simulink model "gm_gmStateSpaceHDL_uz_JL_invModel_ideal"  (R2025a)
settings: Solver=FixedStepDiscrete  StartTime=0.0  StopTime=0.1  RelTol=1e-3
InitFcn:
  | load('C:\Users\jonat\Nextcloud\Ohm\ELSYS\MA_Jonathan_Link\Simulink\sschdl\uz_JL_invModel_ideal\stateSpaceParameters.mat');
undefined symbols (not defined in the file or in its folder): stateSpaceParameters_1
libraries: hdlmdlgenlib x7, hdlssclib x2
settings Model: Creator=jonat  LastModifiedBy=jonat
settings SolverCC: AlgebraicLoopSolver=TrustRegion
settings DataIOCC: LimitDataPoints=on  SaveOutput=off  SaveTime=off
settings OptimizationCC: BlockReduction=off  ConditionallyExecuteInputs=off  DefaultParameterBehavior=Inlined  InheritOutputTypeSmallerThanSingle=on  LifeSpan=inf
settings DebuggingCC: AlgebraicLoopMsg=error  InheritedTsInSrcMsg=none  SingleTaskRateTransMsg=error  UnconnectedInputMsg=warning  UnconnectedOutputMsg=warning  UnconnectedLineMsg=warning  AllowSymbolicDim=off  StrictBusMsg=ErrorOnBusTreatedAsVector  SFUnexpectedBacktrackingDiag=warning  SFNoUnconditionalDefaultTransitionDiag=warning  SFExecutionAtInitializationDiag=none  ArithmeticOperatorsInVariantConditions=warning
settings HardwareCC: ProdBitPerPointer=32.0  ProdBitPerSizeT=32.0  ProdBitPerPtrDiffT=32.0  ProdLargestAtomicFloat=None  ProdIntDivRoundTo=Undefined  ProdEndianess=Unspecified  ProdWordSize=32.0  ProdHWDeviceType=ASIC/FPGA->ASIC/FPGA  ProdEqTarget=off
settings ModelReferenceCC: EnableRefExpFcnMdlSchedulingChecks=on
settings SFSimCC: SimUseLocalCustomCode=off  CustomCodeUndefinedFunction=UseInterfaceOnly
settings RTWCC: RTWUseLocalCustomCode=off  GPUComputeCapability=3.5
settings CodeAppCC: StateflowObjectComments=on
settings GRTTargetCC: TargetLangStandard=C89/C90 (ANSI)
settings ConfigComp: CovScope=ReferencedModels  CovMetricSettings=dw  CovSaveCumulativeToWorkspaceVar=on  CovSaveSingleToWorkspaceVar=on  CovExternalEMLEnable=off  CovSFcnEnable=off

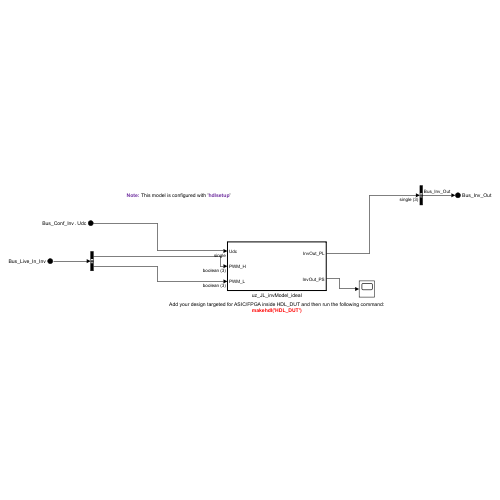
[thumbnail: Simulink's stored preview of the top-level diagram]
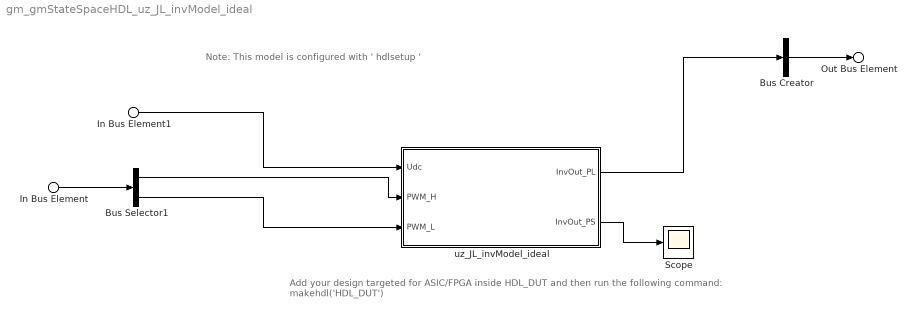
== system gm_gmStateSpaceHDL_uz_JL_invModel_ideal ==
  note: Add your design targeted for ASIC/FPGA inside HDL_DUT and then run the following command:
      | makehdl('HDL_DUT')
  note: Note: This model is configured with ' hdlsetup '
  In Bus Element : Inport  PortName=Bus_Live_In_Inv
  In Bus Element1 : Inport  Port=2  PortName=Bus_Conf_Inv  Element=Udc
  Bus Creator : BusCreator  Inputs=1  OutDataTypeStr=Bus: Bus_Inv_Out  NonVirtualBus=on
      settings: InheritFromInputs=off
  Bus Selector1 : BusSelector  OutputSignals=PWM_H,PWM_L
  Scope : Scope
      settings: ActiveDisplayYMinimum=-497.00837732959218  ActiveDisplayYMaximum=484.07881017040796
  uz_JL_invModel_ideal : Subsystem  TreatAsAtomicUnit=on
  Out Bus Element : Outport  PortName=Bus_Inv_Out
  wires:
  uz_JL_invModel_ideal/1(InvOut_PL) -> Bus Creator/1
  Bus Selector1/2 -> uz_JL_invModel_ideal/3(PWM_L)
  Bus Selector1/1 -> uz_JL_invModel_ideal/2(PWM_H)
  In Bus Element1/1 -> uz_JL_invModel_ideal/1(Udc)
  uz_JL_invModel_ideal/2(InvOut_PS) -> Scope/1
  Bus Creator/1 -> Out Bus Element/1
  In Bus Element/1 -> Bus Selector1/1

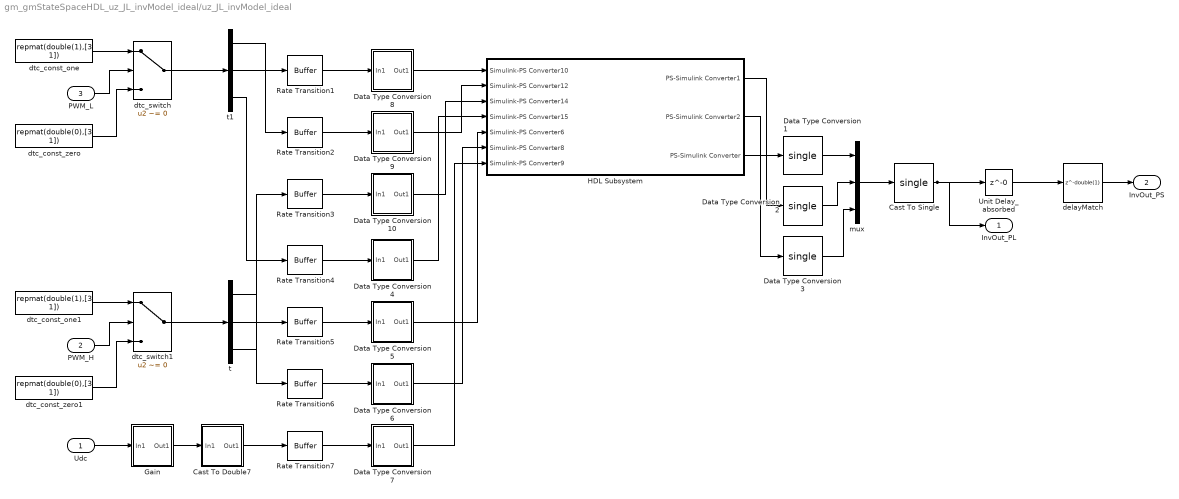
== system gm_gmStateSpaceHDL_uz_JL_invModel_ideal/uz_JL_invModel_ideal ==
  Udc : Inport  OutDataTypeStr=single  PortDimensions=1  SampleTime=1e-08
  PWM_H : Inport  Port=2  OutDataTypeStr=boolean  PortDimensions=[3]  SampleTime=1e-08
  PWM_L : Inport  Port=3  OutDataTypeStr=boolean  PortDimensions=[3]  SampleTime=1e-08
  Cast To Double7 : Subsystem
      mask Display: disp('NFP\nconv');
  Cast To Single : DataTypeConversion  OutDataTypeStr=single
  Data Type Conversion1 : DataTypeConversion  OutDataTypeStr=single
  Data Type Conversion10 : Subsystem
      mask Display: disp('NFP\nconv');
  Data Type Conversion2 : DataTypeConversion  OutDataTypeStr=single
  Data Type Conversion3 : DataTypeConversion  OutDataTypeStr=single
  Data Type Conversion4 : Subsystem
      mask Display: disp('NFP\nconv');
  Data Type Conversion5 : Subsystem
      mask Display: disp('NFP\nconv');
  Data Type Conversion6 : Subsystem
      mask Display: disp('NFP\nconv');
  Data Type Conversion7 : Subsystem
      mask Display: disp('NFP\nconv');
  Data Type Conversion8 : Subsystem
      mask Display: disp('NFP\nconv');
  Data Type Conversion9 : Subsystem
      mask Display: disp('NFP\nconv');
  Gain : Subsystem
      mask Display: disp('NFP\ngain_pow2');
  HDL Subsystem : Subsystem
  Rate Transition{1..7} (7 alike) : hdlmdlgenlib/Buffer
  Unit Delay_absorbed : Delay  DelayLength=0
  delayMatch : Delay  DelayLength=double(1)  InitialCondition=0  SampleTime=1e-08
  dtc_const_one : Constant  Value="repmat(double(1),[3  1])"  OutDataTypeStr=double  SampleTime=1e-08
  dtc_const_one1 : Constant  Value="repmat(double(1),[3  1])"  OutDataTypeStr=double  SampleTime=1e-08
  dtc_const_zero : Constant  Value="repmat(double(0),[3  1])"  OutDataTypeStr=double  SampleTime=1e-08
  dtc_const_zero1 : Constant  Value="repmat(double(0),[3  1])"  OutDataTypeStr=double  SampleTime=1e-08
  dtc_switch : Switch  Criteria=u2 ~= 0  Threshold=double(0)  OutDataTypeStr=double  SampleTime=1e-08  SaturateOnIntegerOverflow=off  InputSameDT=off
  dtc_switch1 : Switch  Criteria=u2 ~= 0  Threshold=double(0)  OutDataTypeStr=double  SampleTime=1e-08  SaturateOnIntegerOverflow=off  InputSameDT=off
  mux : Mux  Inputs=3
  t : Demux  Outputs=3
  t1 : Demux  Outputs=3
  InvOut_PL : Outport  SampleTime=1e-08
  InvOut_PS : Outport  Port=2  SampleTime=1e-08
  wires:
  dtc_const_one/1 -> dtc_switch/1
  dtc_const_one1/1 -> dtc_switch1/1
  delayMatch/1 -> InvOut_PS/1
  PWM_L/1 -> dtc_switch/2
  dtc_const_zero/1 -> dtc_switch/3
  dtc_const_zero1/1 -> dtc_switch1/3
  PWM_H/1 -> dtc_switch1/2
  Data Type Conversion4/1(Out1) -> HDL Subsystem/4(Simulink-PS Converter15)
  Data Type Conversion8/1(Out1) -> HDL Subsystem/1(Simulink-PS Converter10)
  dtc_switch/1 -> t1/1
  Udc/1 -> Gain/1(In1)
  dtc_switch1/1 -> t/1
  Data Type Conversion5/1(Out1) -> HDL Subsystem/5(Simulink-PS Converter6)
  Data Type Conversion9/1(Out1) -> HDL Subsystem/2(Simulink-PS Converter12)
  Gain/1(Out1) -> Cast To Double7/1(In1)
  Data Type Conversion7/1(Out1) -> HDL Subsystem/7(Simulink-PS Converter9)
  Data Type Conversion10/1(Out1) -> HDL Subsystem/3(Simulink-PS Converter14)
  t1/1 -> Rate Transition2/1
  HDL Subsystem/1(PS-Simulink Converter1) -> Data Type Conversion2/1
  t1/2 -> Rate Transition1/1
  t1/3 -> Rate Transition4/1
  t/1 -> Rate Transition6/1
  t/2 -> Rate Transition5/1
  t/3 -> Rate Transition3/1
  Data Type Conversion6/1(Out1) -> HDL Subsystem/6(Simulink-PS Converter8)
  Cast To Double7/1(Out1) -> Rate Transition7/1
  Rate Transition1/1 -> Data Type Conversion8/1(In1)
  Rate Transition2/1 -> Data Type Conversion9/1(In1)
  Rate Transition3/1 -> Data Type Conversion10/1(In1)
  Rate Transition4/1 -> Data Type Conversion4/1(In1)
  Rate Transition5/1 -> Data Type Conversion5/1(In1)
  Rate Transition6/1 -> Data Type Conversion6/1(In1)
  HDL Subsystem/2(PS-Simulink Converter2) -> Data Type Conversion3/1
  Rate Transition7/1 -> Data Type Conversion7/1(In1)
  HDL Subsystem/3(PS-Simulink Converter) -> Data Type Conversion1/1
  Data Type Conversion1/1 -> mux/1
  Data Type Conversion2/1 -> mux/2
  Data Type Conversion3/1 -> mux/3
  mux/1 -> Cast To Single/1
  Unit Delay_absorbed/1 -> delayMatch/1
  Cast To Single/1 -> InvOut_PL/1, Unit Delay_absorbed/1

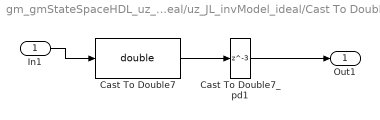
== system gm_gmStateSpaceHDL_uz_JL_invModel_ideal/uz_JL_invModel_ideal/Cast To Double7 ==
  In1 : Inport
  Cast To Double7 : DataTypeConversion  OutDataTypeStr=double  SampleTime=1e-08  SaturateOnIntegerOverflow=off  RndMeth=Floor
  Cast To Double7_pd1 : Delay  DelayLength=3
  Out1 : Outport
  wires:
  In1/1 -> Cast To Double7/1
  Cast To Double7/1 -> Cast To Double7_pd1/1
  Cast To Double7_pd1/1 -> Out1/1

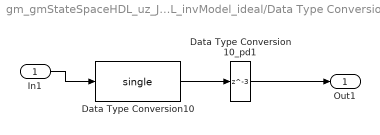
== system gm_gmStateSpaceHDL_uz_JL_invModel_ideal/uz_JL_invModel_ideal/Data Type Conversion10 ==
  In1 : Inport
  Data Type Conversion10 : DataTypeConversion  OutDataTypeStr=single  RndMeth=Nearest  SampleTime=1e-08  SaturateOnIntegerOverflow=off
  Data Type Conversion10_pd1 : Delay  DelayLength=3
  Out1 : Outport
  wires:
  In1/1 -> Data Type Conversion10/1
  Data Type Conversion10/1 -> Data Type Conversion10_pd1/1
  Data Type Conversion10_pd1/1 -> Out1/1

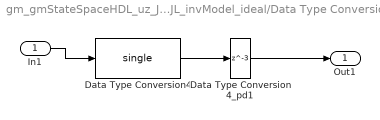
== system gm_gmStateSpaceHDL_uz_JL_invModel_ideal/uz_JL_invModel_ideal/Data Type Conversion4 ==
  In1 : Inport
  Data Type Conversion4 : DataTypeConversion  OutDataTypeStr=single  RndMeth=Nearest  SampleTime=1e-08  SaturateOnIntegerOverflow=off
  Data Type Conversion4_pd1 : Delay  DelayLength=3
  Out1 : Outport
  wires:
  In1/1 -> Data Type Conversion4/1
  Data Type Conversion4/1 -> Data Type Conversion4_pd1/1
  Data Type Conversion4_pd1/1 -> Out1/1

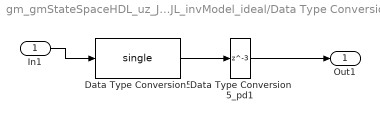
== system gm_gmStateSpaceHDL_uz_JL_invModel_ideal/uz_JL_invModel_ideal/Data Type Conversion5 ==
  In1 : Inport
  Data Type Conversion5 : DataTypeConversion  OutDataTypeStr=single  RndMeth=Nearest  SampleTime=1e-08  SaturateOnIntegerOverflow=off
  Data Type Conversion5_pd1 : Delay  DelayLength=3
  Out1 : Outport
  wires:
  In1/1 -> Data Type Conversion5/1
  Data Type Conversion5/1 -> Data Type Conversion5_pd1/1
  Data Type Conversion5_pd1/1 -> Out1/1

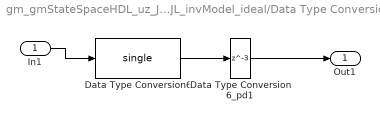
== system gm_gmStateSpaceHDL_uz_JL_invModel_ideal/uz_JL_invModel_ideal/Data Type Conversion6 ==
  In1 : Inport
  Data Type Conversion6 : DataTypeConversion  OutDataTypeStr=single  RndMeth=Nearest  SampleTime=1e-08  SaturateOnIntegerOverflow=off
  Data Type Conversion6_pd1 : Delay  DelayLength=3
  Out1 : Outport
  wires:
  In1/1 -> Data Type Conversion6/1
  Data Type Conversion6/1 -> Data Type Conversion6_pd1/1
  Data Type Conversion6_pd1/1 -> Out1/1

== system gm_gmStateSpaceHDL_uz_JL_invModel_ideal/uz_JL_invModel_ideal/Data Type Conversion7 ==
  In1 : Inport
  Data Type Conversion7 : DataTypeConversion  OutDataTypeStr=single  RndMeth=Nearest  SampleTime=1e-08  SaturateOnIntegerOverflow=off
  Data Type Conversion7_pd1 : Delay  DelayLength=3
  Out1 : Outport
  wires:
  In1/1 -> Data Type Conversion7/1
  Data Type Conversion7/1 -> Data Type Conversion7_pd1/1
  Data Type Conversion7_pd1/1 -> Out1/1

== system gm_gmStateSpaceHDL_uz_JL_invModel_ideal/uz_JL_invModel_ideal/Data Type Conversion8 ==
  In1 : Inport
  Data Type Conversion8 : DataTypeConversion  OutDataTypeStr=single  RndMeth=Nearest  SampleTime=1e-08  SaturateOnIntegerOverflow=off
  Data Type Conversion8_pd1 : Delay  DelayLength=3
  Out1 : Outport
  wires:
  In1/1 -> Data Type Conversion8/1
  Data Type Conversion8/1 -> Data Type Conversion8_pd1/1
  Data Type Conversion8_pd1/1 -> Out1/1

== system gm_gmStateSpaceHDL_uz_JL_invModel_ideal/uz_JL_invModel_ideal/Data Type Conversion9 ==
  In1 : Inport
  Data Type Conversion9 : DataTypeConversion  OutDataTypeStr=single  RndMeth=Nearest  SampleTime=1e-08  SaturateOnIntegerOverflow=off
  Data Type Conversion9_pd1 : Delay  DelayLength=3
  Out1 : Outport
  wires:
  In1/1 -> Data Type Conversion9/1
  Data Type Conversion9/1 -> Data Type Conversion9_pd1/1
  Data Type Conversion9_pd1/1 -> Out1/1

== system gm_gmStateSpaceHDL_uz_JL_invModel_ideal/uz_JL_invModel_ideal/Gain ==
  In1 : Inport
  Gain : Gain  Gain=single(0.5)
  Gain_pd1 : Delay  DelayLength=1
  Out1 : Outport
  wires:
  In1/1 -> Gain/1
  Gain/1 -> Gain_pd1/1
  Gain_pd1/1 -> Out1/1

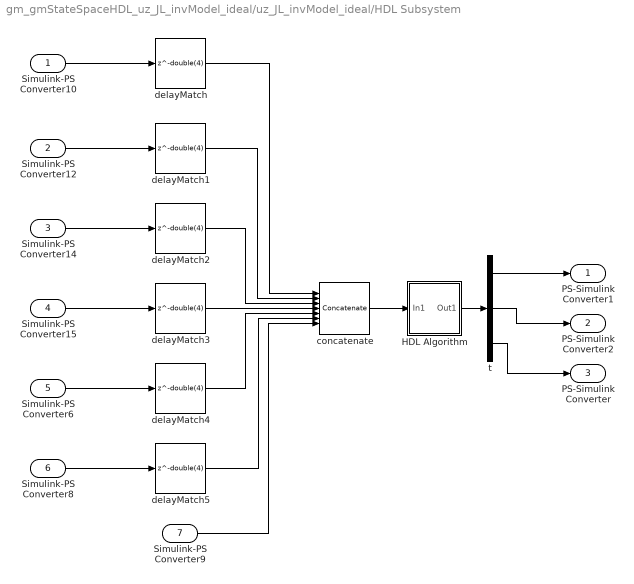
== system gm_gmStateSpaceHDL_uz_JL_invModel_ideal/uz_JL_invModel_ideal/HDL Subsystem ==
  Simulink-PS Converter10 : Inport  OutDataTypeStr=single  PortDimensions=1  SampleTime=1e-08
  Simulink-PS Converter12 : Inport  Port=2  OutDataTypeStr=single  PortDimensions=1  SampleTime=1e-08
  Simulink-PS Converter14 : Inport  Port=3  OutDataTypeStr=single  PortDimensions=1  SampleTime=1e-08
  Simulink-PS Converter15 : Inport  Port=4  OutDataTypeStr=single  PortDimensions=1  SampleTime=1e-08
  Simulink-PS Converter6 : Inport  Port=5  OutDataTypeStr=single  PortDimensions=1  SampleTime=1e-08
  Simulink-PS Converter8 : Inport  Port=6  OutDataTypeStr=single  PortDimensions=1  SampleTime=1e-08
  Simulink-PS Converter9 : Inport  Port=7  OutDataTypeStr=single  PortDimensions=1  SampleTime=1e-08
  HDL Algorithm : Subsystem
  concatenate : Concatenate  NumInputs=7
  delayMatch{,1..5} (6 alike) : Delay  DelayLength=double(4)  InitialCondition=0  SampleTime=1e-08
  t : Demux  Outputs=3
  PS-Simulink Converter1 : Outport  SampleTime=1e-08
  PS-Simulink Converter2 : Outport  Port=2  SampleTime=1e-08
  PS-Simulink Converter : Outport  Port=3  SampleTime=1e-08
  wires:
  Simulink-PS Converter6/1 -> delayMatch4/1
  Simulink-PS Converter10/1 -> delayMatch/1
  Simulink-PS Converter8/1 -> delayMatch5/1
  Simulink-PS Converter12/1 -> delayMatch1/1
  Simulink-PS Converter14/1 -> delayMatch2/1
  t/3 -> PS-Simulink Converter/1
  Simulink-PS Converter15/1 -> delayMatch3/1
  delayMatch/1 -> concatenate/1
  delayMatch1/1 -> concatenate/2
  delayMatch2/1 -> concatenate/3
  delayMatch3/1 -> concatenate/4
  delayMatch4/1 -> concatenate/5
  delayMatch5/1 -> concatenate/6
  Simulink-PS Converter9/1 -> concatenate/7
  t/1 -> PS-Simulink Converter1/1
  concatenate/1 -> HDL Algorithm/1(In1)
  HDL Algorithm/1(Out1) -> t/1
  t/2 -> PS-Simulink Converter2/1

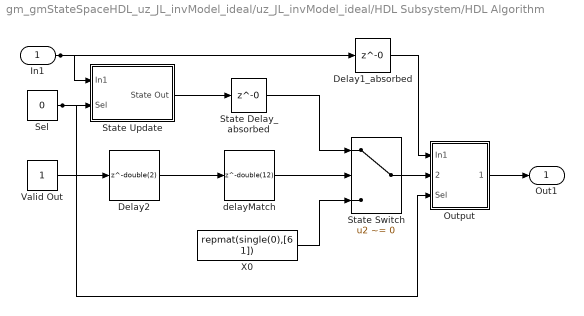
== system gm_gmStateSpaceHDL_uz_JL_invModel_ideal/uz_JL_invModel_ideal/HDL Subsystem/HDL Algorithm ==
  In1 : Inport  OutDataTypeStr=single  PortDimensions=[7]  SampleTime=1e-08
  Delay1_absorbed : Delay  DelayLength=0
  Delay2 : Delay  DelayLength=double(2)  InitialCondition=0  SampleTime=1e-08
  Output : Subsystem
  Sel : Constant  Value=0  OutDataTypeStr=uint32  SampleTime=1e-08
  State Delay_absorbed : Delay  DelayLength=0
  State Switch : Switch  Criteria=u2 ~= 0  Threshold="fi(0,0,1,0,\"hex\",\"0\")"  OutDataTypeStr=single  SampleTime=1e-08  SaturateOnIntegerOverflow=off  InputSameDT=off
  State Update : Subsystem
  Valid Out : Constant  OutDataTypeStr=boolean  SampleTime=1e-08
  X0 : Constant  Value="repmat(single(0),[6  1])"  OutDataTypeStr=single  SampleTime=1e-08
  delayMatch : Delay  DelayLength=double(12)  InitialCondition=0  SampleTime=1e-08
  Out1 : Outport  SampleTime=1e-08  VectorParamsAs1DForOutWhenUnconnected=off
  wires:
  In1/1 -> Delay1_absorbed/1, State Update/1(In1)
  X0/1 -> State Switch/3
  delayMatch/1 -> State Switch/2
  Sel/1 -> Output/3(Sel), State Update/2(Sel)
  State Delay_absorbed/1 -> State Switch/1
  Valid Out/1 -> Delay2/1
  State Update/1(State Out) -> State Delay_absorbed/1
  Delay2/1 -> delayMatch/1
  Delay1_absorbed/1 -> Output/1(In1)
  State Switch/1 -> Output/2(State)
  Output/1(Out1) -> Out1/1

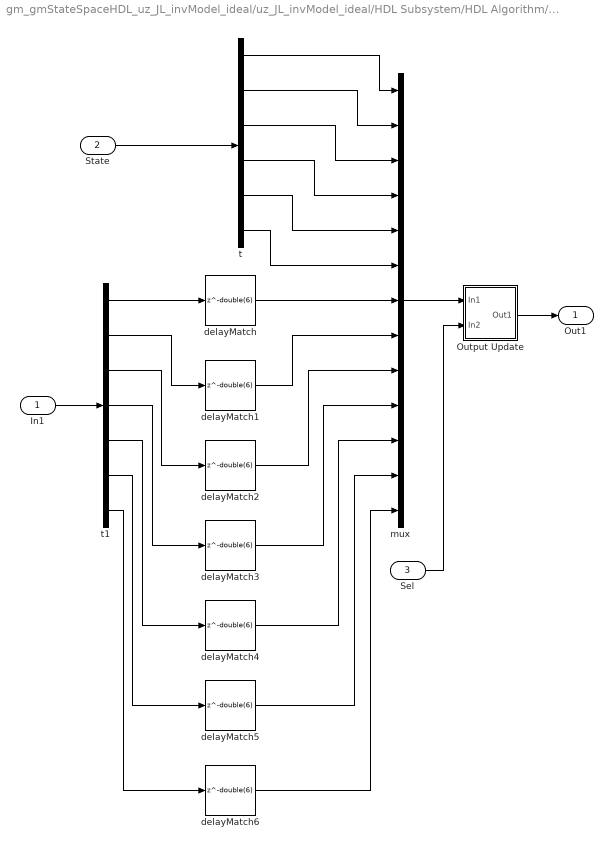
== system gm_gmStateSpaceHDL_uz_JL_invModel_ideal/uz_JL_invModel_ideal/HDL Subsystem/HDL Algorithm/Output ==
  In1 : Inport  OutDataTypeStr=single  PortDimensions=[7]  SampleTime=1e-08
  State : Inport  Port=2  OutDataTypeStr=single  PortDimensions=[6]  SampleTime=1e-08
  Sel : Inport  Port=3  OutDataTypeStr=uint32  PortDimensions=1  SampleTime=1e-08  LockScale=on
  Output Update : Subsystem
  delayMatch{,1..6} (7 alike) : Delay  DelayLength=double(6)  InitialCondition=0  SampleTime=1e-08
  mux : Mux  Inputs=13
  t : Demux  Outputs=6
  t1 : Demux  Outputs=7
  Out1 : Outport  SampleTime=1e-08  VectorParamsAs1DForOutWhenUnconnected=off
  wires:
  In1/1 -> t1/1
  State/1 -> t/1
  t1/5 -> delayMatch4/1
  t1/3 -> delayMatch2/1
  t1/1 -> delayMatch/1
  t1/6 -> delayMatch5/1
  t1/4 -> delayMatch3/1
  t1/2 -> delayMatch1/1
  t1/7 -> delayMatch6/1
  t/1 -> mux/1
  t/2 -> mux/2
  t/3 -> mux/3
  t/4 -> mux/4
  mux/1 -> Output Update/1(In1)
  t/5 -> mux/5
  t/6 -> mux/6
  delayMatch/1 -> mux/7
  delayMatch1/1 -> mux/8
  delayMatch2/1 -> mux/9
  delayMatch3/1 -> mux/10
  delayMatch4/1 -> mux/11
  Sel/1 -> Output Update/2(In2)
  delayMatch5/1 -> mux/12
  delayMatch6/1 -> mux/13
  Output Update/1(Out1) -> Out1/1

== system gm_gmStateSpaceHDL_uz_JL_invModel_ideal/uz_JL_invModel_ideal/HDL Subsystem/HDL Algorithm/State Update ==
  In1 : Inport  OutDataTypeStr=single  PortDimensions=[7]  SampleTime=1e-08
  Sel : Inport  Port=2  OutDataTypeStr=uint32  PortDimensions=1  SampleTime=1e-08  LockScale=on
  State Update : Subsystem
  State Out : Outport  OutDataTypeStr=single  SampleTime=1e-08  VectorParamsAs1DForOutWhenUnconnected=off
  wires:
  In1/1 -> State Update/1(In1)
  Sel/1 -> State Update/2(In2)
  State Update/1(Out1) -> State Out/1

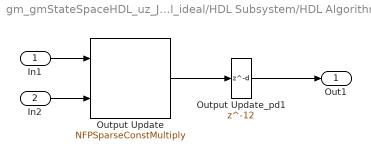
== system gm_gmStateSpaceHDL_uz_JL_invModel_ideal/uz_JL_invModel_ideal/HDL Subsystem/HDL Algorithm/Output/Output Update ==
  In1 : Inport
  In2 : Inport  Port=2
  Output Update : hdlssclib/NFPSparseConstMultiply  MatrixSource=Dialog  constMatrix=single([stateSpaceParameters_1.Cd stateSpaceParameters_1.Dd])  MatrixType=single  MatrixSize=[1 1]  ColumnIndices=[1]  RowIndices=[1]  PropDataType=single  defWL=48
  Output Update_pd1 : Delay  DelayLength=12
  Out1 : Outport
  wires:
  Output Update_pd1/1 -> Out1/1
  In1/1 -> Output Update/1
  Output Update/1 -> Output Update_pd1/1
  In2/1 -> Output Update/2

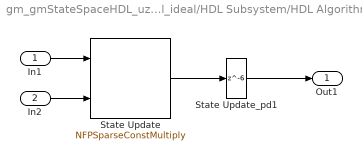
== system gm_gmStateSpaceHDL_uz_JL_invModel_ideal/uz_JL_invModel_ideal/HDL Subsystem/HDL Algorithm/State Update/State Update ==
  In1 : Inport
  In2 : Inport  Port=2
  State Update : hdlssclib/NFPSparseConstMultiply  MatrixSource=Dialog  constMatrix=single([ stateSpaceParameters_1.Bd])  MatrixType=single  MatrixSize=[1 1]  ColumnIndices=[1]  RowIndices=[1]  PropDataType=single  defWL=48
  State Update_pd1 : Delay  DelayLength=6
  Out1 : Outport
  wires:
  In1/1 -> State Update/1
  In2/1 -> State Update/2
  State Update/1 -> State Update_pd1/1
  State Update_pd1/1 -> Out1/1
